simulink model "tuning_PID"  (R2020b)
settings: Solver=ode4  StartTime=0.0  StopTime=10  MaxStep=0.2  RelTol=1e-3
undefined symbols (not defined in the file): k
settings Model: Creator=K E S SRINIVAS  LastModifiedBy=K E S SRINIVAS
settings DataIOCC: ReturnWorkspaceOutputs=off

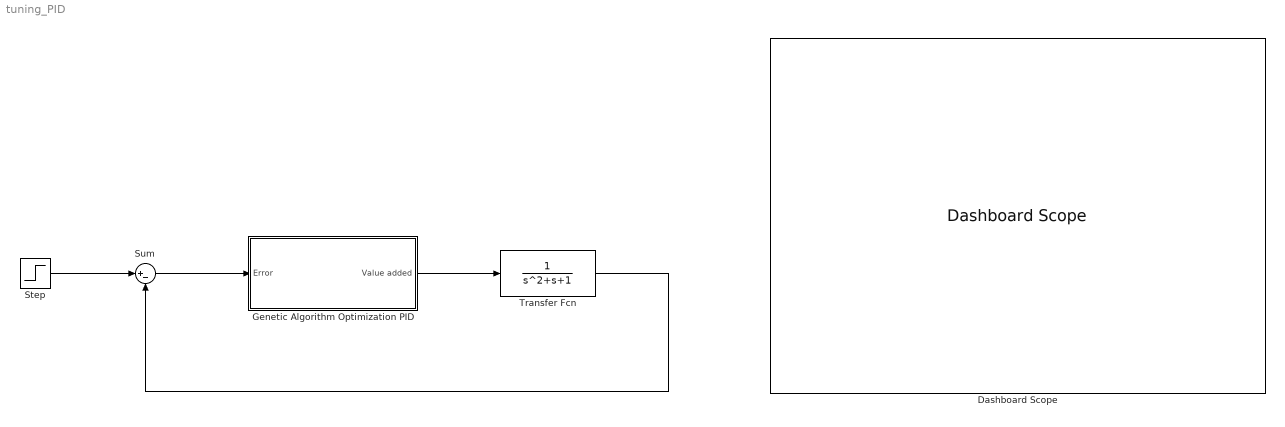
== system tuning_PID ==
  Dashboard Scope : DashboardScope
  Genetic Algorithm Optimization PID : Subsystem
  Step : Step  SampleTime=0
  Sum : Sum  Inputs=|+-
  Transfer Fcn : TransferFcn  Denominator=[1 1 1]
  wires:
  Transfer Fcn/1 -> Sum/2
  Step/1 -> Sum/1
  Sum/1 -> Genetic Algorithm Optimization PID/1(Error)
  Genetic Algorithm Optimization PID/1(Value added) -> Transfer Fcn/1

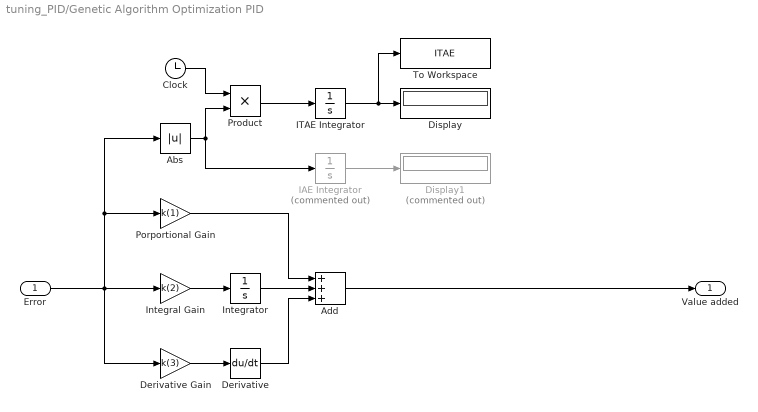
== system tuning_PID/Genetic Algorithm Optimization PID ==
  Error : Inport
  Abs : Abs
  Add : Sum  Inputs=+++
  Clock : Clock
  Derivative : Derivative
  Derivative Gain : Gain  Gain=k(3)
  Display : Display
  Display1 : Display  Commented=on
  IAE Integrator : Integrator  Commented=on
  ITAE Integrator : Integrator
  Integral Gain : Gain  Gain=k(2)
  Integrator : Integrator
  Porportional Gain : Gain  Gain=k(1)
  Product : Product
  To Workspace : ToWorkspace  VariableName=ITAE  SampleTime=-1
  Value added : Outport
  wires:
  Error/1 -> Abs/1, Porportional Gain/1, Derivative Gain/1, Integral Gain/1
  Abs/1 -> IAE Integrator/1, Product/2
  Clock/1 -> Product/1
  IAE Integrator/1 -> Display1/1
  Derivative Gain/1 -> Derivative/1
  Integrator/1 -> Add/2
  Porportional Gain/1 -> Add/1
  Derivative/1 -> Add/3
  Integral Gain/1 -> Integrator/1
  ITAE Integrator/1 -> To Workspace/1, Display/1
  Product/1 -> ITAE Integrator/1
  Add/1 -> Value added/1
